simulink model "HeartModelECG2"  (R2014a)
settings: Solver=FixedStepDiscrete  StartTime=0.0  StopTime=60  FixedStep=0.001  RelTol=1e-3
values from neighbouring files (symbols this model uses):
  Atr_refrD = 50    [matlab.mat]
  AV_alpha = 150    [matlab.mat]
  AV_anteDMin = 100    [matlab.mat]
  AV_beta = 250    [matlab.mat]
  AV_delta = 10    [matlab.mat]
  AV_k4 = 0.03    [matlab.mat]
  AV_refrDMin = 50    [matlab.mat]
  AV_retroDMin = 100    [matlab.mat]
  AV_tauC = 100    [matlab.mat]
  AV_theta = 10    [matlab.mat]
  AV_tr = 500    [matlab.mat]
  AV_Vr = -90    [matlab.mat]
  AV_Vt = -40    [matlab.mat]
  ParECG = [14.7251920614 -18.4251553773 187.03806143 -54.3910305813 76.7618958079 0.0484383561644 0.0300821917808 0.0317260273973 0.0682739726027 0.081698630137 1 1 ... (15 elements, 5x3)]    [matlab.mat]
  PM_TAVI = 150    [matlab.mat]
  PM_TLRI = 1000    [matlab.mat]
  PM_TPVAB = 50    [matlab.mat]
  PM_TPVARP = 250    [matlab.mat]
  PM_TURI = 400    [matlab.mat]
  PM_TVRP = 320    [matlab.mat]
  RA_anteD = 75.8904109589    [matlab.mat]
  RA_retroD = 30    [matlab.mat]
  RV_anteD = 50    [matlab.mat]
  RV_retroD = 50    [matlab.mat]
  SA_dV = 50    [matlab.mat]
  SA_ectopD = 10400    [matlab.mat]
  SA_ectopdV = 50    [matlab.mat]
  SA_noiseD = 1000000    [matlab.mat]
  VRG_d = 3000    [matlab.mat]
  VRG_ectopD = 30450    [matlab.mat]
  VRG_noiseD = 1000000    [matlab.mat]
  Vtr_refrD = 252.054794521    [matlab.mat]
libraries: simulink x4
settings Model: Creator=alexandru  LastModifiedBy=paoletti
settings SolverCC: AlgebraicLoopSolver=LineSearch
settings DataIOCC: LimitDataPoints=off  SignalLogging=off  DSMLogging=off  SaveTime=off
settings HardwareCC: TargetBitPerLong=64  TargetBitPerPointer=64  TargetLongLongMode=on  TargetIntDivRoundTo=Zero  TargetEndianess=LittleEndian  TargetWordSize=64  TargetHWDeviceType=MATLAB Host  ProdEqTarget=off
settings RTWCC: SystemTargetFile=rsim.tlc  GenCodeOnly=on  PackageGeneratedCodeAndArtifacts=on  PackageName=idhp_model_heart_realtime  TemplateMakefile=rsim_default_tmf  Description=Rapid Simulation Target  ProcessScript=rsim_make_rtw_hook
settings RSimTargetCC: ERTMultiwordTypeDef=System defined  ERTMultiwordLength=256  EnableShiftOperators=on

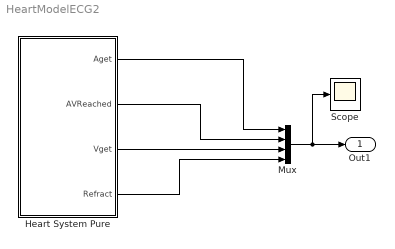
== system HeartModelECG2 ==
  Heart System Pure : Subsystem
  Mux : Mux
  Scope : Scope
  Out1 : Outport
  wires:
  Mux/1 -> Scope/1, Out1/1
  Heart System Pure/2(AVReached) -> Mux/2
  Heart System Pure/3(Vget) -> Mux/3
  Heart System Pure/4(Refract) -> Mux/4
  Heart System Pure/1(Aget) -> Mux/1

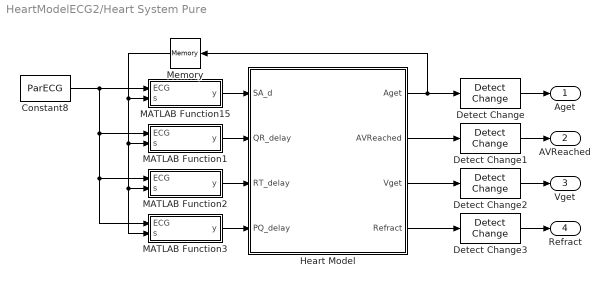
== system HeartModelECG2/Heart System Pure ==
  Constant8 : Constant  Value=ParECG
  Detect Change{,1..3} (4 alike) : simulink/Logic and Bit Operations/Detect Change  vinit=0  InputProcessing=Inherited  OutDataTypeStr=boolean
  Heart Model : Stateflow chart  Priority=1  TreatAsAtomicUnit=on
  MATLAB Function1 : MATLAB Function  TreatAsAtomicUnit=on
  MATLAB Function15 : MATLAB Function  TreatAsAtomicUnit=on
  MATLAB Function2 : MATLAB Function  TreatAsAtomicUnit=on
  MATLAB Function3 : MATLAB Function  TreatAsAtomicUnit=on
  Memory : Memory
  Aget : Outport
  AVReached : Outport  Port=2
  Vget : Outport  Port=3
  Refract : Outport  Port=4
  wires:
  MATLAB Function15/1(y) -> Heart Model/1(SA_d)
  MATLAB Function1/1(y) -> Heart Model/2(QR_delay)
  MATLAB Function2/1(y) -> Heart Model/3(RT_delay)
  MATLAB Function3/1(y) -> Heart Model/4(PQ_delay)
  Constant8/1 -> MATLAB Function3/1(ECG), MATLAB Function2/1(ECG), MATLAB Function1/1(ECG), MATLAB Function15/1(ECG)
  Heart Model/1(Aget) -> Memory/1, Detect Change/1
  Heart Model/2(AVReached) -> Detect Change1/1
  Heart Model/3(Vget) -> Detect Change2/1
  Heart Model/4(Refract) -> Detect Change3/1
  Memory/1 -> MATLAB Function1/2(s), MATLAB Function2/2(s), MATLAB Function3/2(s), MATLAB Function15/2(s)
  Detect Change/1 -> Aget/1
  Detect Change1/1 -> AVReached/1
  Detect Change2/1 -> Vget/1
  Detect Change3/1 -> Refract/1

== matlab function HeartModelECG2/Heart System Pure/MATLAB Function15 ==
  data: y output; ECG input; s input
function y = fcn(ECG,s)
persistent e;
persistent os;

if (isempty(os))
    os = false;
end
    
if (isempty(e) || s~=os) 
    r = unidrnd(size(ECG,1),1,1);
    e = ECG(r,11);
    os = s;
end   
y = e;

== stateflow chart HeartModelECG2/Heart System Pure/Heart Model ==
  settings: updateMethod=DISCRETE  sampleTime=0.001
  state Heart
    state A_dV [parallel]
      settings: executionOrder=13
      state a_dVLow
      state a_dvHigh
      (default) -> a_dVLow
      a_dVLow -> a_dvHigh [order 1] : a_dVSetHigh
      a_dVLow -> a_dVLow [order 2] : tr_AVJ
          | {send(AVJAnteReached,AVJ);
          | send(AVReached);}
      a_dvHigh -> a_dvHigh [order 2] : tr_AVJ
          | {send(AVJAnteReachedHigh,AVJ);
          | send(AVReached);}
      a_dvHigh -> a_dVLow [order 1] : a_dVSetLow
    state SANodeEctopic [parallel]
      settings: executionOrder=2
      state q0
      (default) -> Heart.SANodeEctopic.q0
      Heart.SANodeEctopic.q0 -> Heart.SANodeEctopic.q0 : after(SA_ectopD, msec)
          | {send(Abeat,Atrium);
          | send(a_dVSetHigh,A_dV);}
    state AtrNoiseGenerator [parallel]
      settings: executionOrder=1
      state q0
      (default) -> Heart.AtrNoiseGenerator.q0
      Heart.AtrNoiseGenerator.q0 -> Heart.AtrNoiseGenerator.q0 : after(SA_noiseD, msec)
          | {send(Aget);}
    state RAConductor [parallel]
      settings: executionOrder=6
      state Empty
      state Ante
      state Retro
      (default) -> Heart.RAConductor.Empty
      Heart.RAConductor.Empty -> Heart.RAConductor.Ante [order 1] : arg
      Heart.RAConductor.Ante -> Heart.RAConductor.Empty [order 1] : retroAVJ
      Heart.RAConductor.Empty -> Heart.RAConductor.Retro [order 2] : retroAVJ
      Heart.RAConductor.Retro -> Heart.RAConductor.Empty [order 1] : arg
      Heart.RAConductor.Retro -> Heart.RAConductor.Empty [order 2] : after(RA_retroD,msec)
          | {send(AtrRetroReached,...
          | Atrium);}
      Heart.RAConductor.Ante -> Heart.RAConductor.Empty [order 2] : after(PQ_delay,msec)
          | {send(tr_AVJ,A_dV);}
    state AVJOut [parallel]
      settings: executionOrder=4
      state Empty
      state Ante
      state Retro
      (default) -> Heart.AVJOut.Empty
      Heart.AVJOut.Ante -> Heart.AVJOut.Empty : after(AVJDelay(avj_tRec,...
          | QR_delay*0.666),msec)
          | {send(anteAVJ,RVConductor);}
      Heart.AVJOut.Empty -> Heart.AVJOut.Ante [order 1] : AVJAnteExit
      Heart.AVJOut.Retro -> Heart.AVJOut.Empty : after(AVJDelay(avj_tRec,...
          | AV_retroDMin),msec)
          | {send(retroAVJ,...
          | RAConductor);}
      Heart.AVJOut.Empty -> Heart.AVJOut.Retro [order 2] : AVJRetroExit
    state VRGEctopic [parallel]
      settings: executionOrder=10
      state q0
      (default) -> Heart.VRGEctopic.q0
      Heart.VRGEctopic.q0 -> Heart.VRGEctopic.q0 : after(VRG_ectopD, msec)
          | {send(Vbeat,Ventricle);}
    state RVConductor [parallel]
      settings: executionOrder=5
      state Empty
      state Ante
      state Retro
      (default) -> Heart.RVConductor.Empty
      Heart.RVConductor.Empty -> Heart.RVConductor.Ante [order 1] : anteAVJ
      Heart.RVConductor.Empty -> Heart.RVConductor.Retro [order 2] : vrg
      Heart.RVConductor.Ante -> Heart.RVConductor.Empty [order 1] : vrg
      Heart.RVConductor.Ante -> Heart.RVConductor.Empty [order 2] : after(QR_delay/3,msec)
          | {send(VtrAnteReached,...
          | Ventricle);}
      Heart.RVConductor.Retro -> Heart.RVConductor.Empty [order 1] : anteAVJ
      Heart.RVConductor.Retro -> Heart.RVConductor.Empty [order 2] : after(RV_retroD,msec)
          | {send(AVJRetroReached,...
          | AVJ);}
    state VtrNoiseGenerator [parallel]
      settings: executionOrder=3
      state q0
      Heart.VtrNoiseGenerator.q0 -> Heart.VtrNoiseGenerator.q0 : after(VRG_noiseD, msec)
          | {send(Vget);}
      (default) -> Heart.VtrNoiseGenerator.q0
    state SANode [parallel]
      settings: executionOrder=7
      state Wait4ABeat
      state Wait4ASynch
      (default) -> Wait4ABeat
      Wait4ABeat -> Wait4ASynch [order 2] : after(SA_d, msec)
          | {send(Abeat,Atrium);
          | send(a_dVSetLow,A_dV);
          | }
      Wait4ABeat -> Wait4ABeat [order 1] : NextAtrBeat
      Wait4ASynch -> Wait4ABeat : NextAtrBeat
    state VRG [parallel]
      settings: executionOrder=11
      state Wait4VBeat
      state Wait4VSynch
      (default) -> Wait4VBeat
      Wait4VBeat -> Wait4VSynch [order 2] : after(VRG_d, msec)
          | {send(Vbeat,Ventricle);}
      Wait4VSynch -> Wait4VBeat : NextVtrBeat
      Wait4VBeat -> Wait4VBeat [order 1] : NextVtrBeat
    state AVJ [parallel]
      settings: executionOrder=12
      state Recovery
      state Ante
      state Refractory
      state Retro
      (default) -> Recovery : {avj_t4=timeToDep(AV_Vr);
          | ctime=0;
          | recoverylast=0;
          | refractorylast=0;
          | }
      Heart.AVJ.Ante -> Heart.AVJ.Refractory : after(avj_t4,msec)
          | {ctime=ctime+temporalCount(msec);
          | avj_tRec=(ctime-recoverylast);
          | send(AVJAnteExit,AVJOut);
          | avj_refr_0=initRefrPeriod(avj_tRec);
          | avj_refr=avj_refr_0;
          | refractorylast=ctime;}
      Recovery -> Heart.AVJ.Ante [order 1] : AVJAnteReached{
          | ctime=ctime+temporalCount(msec);
          | avj_t4 = timeToDep(AV_Vr+ ...
          | (ctime-recoverylast)*AV_k4 + SA_dV);
          | }
      Recovery -> Heart.AVJ.Ante [order 3] : AVJAnteReachedHigh{
          | ctime=ctime+temporalCount(msec);
          | avj_t4 = timeToDep(AV_Vr+...
          | (ctime-recoverylast)*AV_k4 + SA_ectopdV);
          | }
      Heart.AVJ.Refractory -> Recovery [order 4] : after(avj_refr,msec){
          | ctime=ctime+temporalCount(msec);
          | avj_t4=timeToDep(AV_Vr);
          | recoverylast=ctime;
          | }
      Recovery -> Heart.AVJ.Retro [order 4] : AVJRetroReached{
          | ctime=ctime+temporalCount(msec);
          | }
      Recovery -> Heart.AVJ.Refractory [order 2] : after(avj_t4,msec){
          | ctime=ctime+temporalCount(msec);
          | avj_tRec=avj_t4;
          | avj_refr_0=initRefrPeriod(avj_tRec);
          | avj_refr=avj_refr_0;
          | refractorylast=ctime;}
      Heart.AVJ.Refractory -> Heart.AVJ.Refractory [order 3] : AVJAnteReachedHigh
          | {ctime=ctime+temporalCount(msec);
          | avj_refr=avj_refr-(ctime - refractorylast)+...
          | modulateRefrAnte((ctime - refractorylast),...
          | avj_refr_0,SA_ectopdV);
          | refractorylast=ctime;
          | }
      Heart.AVJ.Refractory -> Heart.AVJ.Refractory [order 1] : AVJAnteReached
          | {ctime=ctime+temporalCount(msec);
          | avj_refr=avj_refr-(ctime - refractorylast)+...
          | modulateRefrAnte((ctime - refractorylast),...
          | avj_refr_0,SA_dV);
          | refractorylast=ctime;}
      Heart.AVJ.Refractory -> Heart.AVJ.Refractory [order 2] : AVJRetroReached
          | {ctime=ctime+temporalCount(msec);
          | avj_refr=avj_refr-(ctime - refractorylast)+...
          | modulateRefrRetro((ctime - refractorylast),...
          | avj_refr_0);
          | refractorylast=ctime;}
      Heart.AVJ.Retro -> Heart.AVJ.Refractory : {send(AVJRetroExit,AVJOut);
          | ctime=ctime+temporalCount(msec);
          | avj_tRec=ctime-recoverylast;
          | avj_refr_0=initRefrPeriod(avj_tRec);
          | avj_refr=avj_refr_0;
          | refractorylast=ctime;
          | }
    state Ventricle [parallel]
      settings: executionOrder=8
      state Excitable
      state Refractory
      state VsenseAnte
      state VSynch
      state Vsense
      state GenerateRetroWave
      (default) -> Heart.Ventricle.Refractory
      Heart.Ventricle.Refractory -> Heart.Ventricle.Excitable : after(RT_delay,msec){
          | send(Refract);}
      Heart.Ventricle.Excitable -> Vsense [order 3] : Vbeat
      Heart.Ventricle.Excitable -> VsenseAnte [order 1] : VtrAnteReached
      VSynch -> Heart.Ventricle.Refractory : {send(NextVtrBeat,...
          | VRG);}
      Heart.Ventricle.Excitable -> GenerateRetroWave [order 2] : VP
      VsenseAnte -> VSynch : {send(Vget);}
      GenerateRetroWave -> VSynch : {send(vrg,RVConductor);}
      Vsense -> GenerateRetroWave : {send(Vget);}
    state Atrium [parallel]
      settings: executionOrder=9
      state Excitable
      state Refractory
      state ASynch
      state AsenseRetro
      state Asense
      state GenerateAnteWave
      (default) -> Heart.Atrium.Refractory
      Heart.Atrium.Excitable -> Asense [order 1] : Abeat
      Heart.Atrium.Refractory -> Heart.Atrium.Excitable : after(Atr_refrD,msec)
      Heart.Atrium.Excitable -> AsenseRetro [order 3] : AtrRetroReached
      ASynch -> Heart.Atrium.Refractory : {send(NextAtrBeat,...
          | SANode);}
      Heart.Atrium.Excitable -> GenerateAnteWave [order 2] : AP
      AsenseRetro -> ASynch : {send(Aget);}
      GenerateAnteWave -> ASynch : {send(arg,RAConductor);}
      Asense -> GenerateAnteWave : {send(Aget);}
  (default) -> Heart
  data: t function_output double; tRec function_input double; minDly function_input double; t function_output double; Vm function_input double; t function_output double; tRec function_input double; t function_input double; dT function_output double; t0 function_input double; t function_input double; t0 function_input double; dT function_output double; dV function_input double; Atr_refrD parameter; AV_alpha parameter; AV_anteDMin parameter; AV_beta parameter; AV_delta parameter; AV_k4 parameter; AV_refrDMin parameter; AV_retroDMin parameter; AV_tauC parameter; AV_theta parameter; AV_tr parameter; AV_Vr parameter; AV_Vt parameter; RA_anteD parameter; RA_retroD parameter; RV_anteD parameter; RV_retroD parameter; SA_d input; SA_dV parameter; SA_ectopD parameter; SA_ectopdV parameter; SA_noiseD parameter; VRG_d parameter; VRG_ectopD parameter; VRG_noiseD parameter; Vtr_refrD parameter; avj_tRec local double; clk local double; PM_TAVI parameter; PM_TLRI parameter; PM_TPVAB parameter; PM_TPVARP parameter; PM_TURI parameter; PM_TVRP parameter; recoverylast local double; avj_t4 local double; ctime local double; avj_refr local double; avj_refr_0 local double; refractorylast local double; QR_delay input double; RT_delay input double; PQ_delay input double
  events: Abeat local FUNCTION_CALL_EVENT; AtrRetroReached local FUNCTION_CALL_EVENT; arg local FUNCTION_CALL_EVENT; retroAVJ local FUNCTION_CALL_EVENT; AVJAnteReached local FUNCTION_CALL_EVENT; NextAtrBeat local FUNCTION_CALL_EVENT; AVJRetroReached local FUNCTION_CALL_EVENT; anteAVJ local FUNCTION_CALL_EVENT; vrg local FUNCTION_CALL_EVENT; VtrAnteReached local FUNCTION_CALL_EVENT; AVJRetroExit local FUNCTION_CALL_EVENT; AVJAnteExit local FUNCTION_CALL_EVENT; NextVtrBeat local FUNCTION_CALL_EVENT; Vbeat local FUNCTION_CALL_EVENT; AP local EITHER_EDGE_EVENT; VP local EITHER_EDGE_EVENT; AS local RISING_EDGE_EVENT; VS local RISING_EDGE_EVENT; Aintrinsic local EITHER_EDGE_EVENT; Anoise local EITHER_EDGE_EVENT; Aretro local EITHER_EDGE_EVENT; Vintrinsic local EITHER_EDGE_EVENT; Vnoise local EITHER_EDGE_EVENT; Vante local EITHER_EDGE_EVENT; APElectr local RISING_EDGE_EVENT; VPElectr local EITHER_EDGE_EVENT; IncrClk local FUNCTION_CALL_EVENT; State local FUNCTION_CALL_EVENT; Clk0 local FUNCTION_CALL_EVENT; Clk1 local FUNCTION_CALL_EVENT; a_dVSetHigh local FUNCTION_CALL_EVENT; a_dVSetLow local FUNCTION_CALL_EVENT; tr_AVJ local FUNCTION_CALL_EVENT; AVJAnteReachedHigh local FUNCTION_CALL_EVENT; RLRI local FUNCTION_CALL_EVENT; TAVI local FUNCTION_CALL_EVENT; RTAVI local FUNCTION_CALL_EVENT; RURI local FUNCTION_CALL_EVENT; Aget output EITHER_EDGE_EVENT; AVReached output EITHER_EDGE_EVENT; Vget output EITHER_EDGE_EVENT; Refract output EITHER_EDGE_EVENT
  function t  = AVJDelay(tRec,minDly):
    | function t  = AVJDelay(tRec,minDly)
    |     t = minDly+AV_alpha*exp(-tRec/AV_tauC);
    | end
  function t  = timeToDep(Vm):
    | function t  = timeToDep(Vm)
    |     t = max(0,(AV_Vt-Vm)/AV_k4);
    | end
  function t  = initRefrPeriod(tRec):
    | function t  = initRefrPeriod(tRec)
    |     t = AV_refrDMin + AV_beta*(1 - exp(-tRec/AV_tr));
    | end
  function dT  = modulateRefrRetro(t,t0):
    | 
    | function dT  = modulateRefrRetro(t,t0)
    |     dT = AV_refrDMin*power(t/t0,AV_theta);
    | end
  function dT  = modulateRefrAnte(t,t0,dV):
    | function dT  = modulateRefrAnte(t,t0,dV)
    |     %val1 = t/t0;
    |     %val2 = power(t/t0,avj_theta);
    |     dT = AV_refrDMin*power(t/t0,AV_theta)*power(min(1,dV/(AV_Vt-AV_Vr)),AV_delta);
    |     %fprintf(1,'%f %f\n', val1, val2);
    | end

== matlab function HeartModelECG2/Heart System Pure/MATLAB Function1 ==
  data: y output; ECG input; s input
function y = fcn(ECG,s)
persistent e;
persistent os;

if (isempty(os))
    os = false;
end
    
if (isempty(e) || s~=os) 
    r = unidrnd(size(ECG,1),1,1);
    e = ECG(r,13);
    os = s;
end   
y = e;

== matlab function HeartModelECG2/Heart System Pure/MATLAB Function2 ==
  data: y output; ECG input; s input
function y = fcn(ECG,s)
persistent e;
persistent os;

if (isempty(os))
    os = false;
end
    
if (isempty(e) || s~=os) 
    r = unidrnd(size(ECG,1),1,1);
    e = ECG(r,15);
    os = s;
end   
y = e;

== matlab function HeartModelECG2/Heart System Pure/MATLAB Function3 ==
  data: y output; ECG input; s input
function y = fcn(ECG,s)
persistent e;
persistent os;

if (isempty(os))
    os = false;
end
    
if (isempty(e) || s~=os) 
    r = unidrnd(size(ECG,1),1,1);
    e = ECG(r,12);
    os = s;
end   
y = e;
